simulink model "sf_cruise_control"  (Simulink 6.0)
settings: Solver=ode5  SolverMode=SingleTasking  StartTime=0.0  StopTime=inf  FixedStep=0.005  RelTol=1e-3
PreLoadFcn:
  | Kp = 30; Ki = 10; Kd = 30;
undefined symbols (not defined in the file or in its folder): DiscIntNeverNeededParam
libraries: simulink x1
CloseFcn:
  | figH = findobj('Tag','sf_cruise_control_ui'); if ~isempty(figH) delete(figH); end
settings Model: CovMetricSettings=dcmtr  CovHTMLOptions=-aTS=0 -bRG=1 -bTC=0 -hTR=0 -nFC=1  Creator=The MathWorks Inc.  LastModifiedBy=batserve  ExtModeAutoUpdateStatusClock=off
settings OptimizationCC: BooleanDataType=off
settings DebuggingCC: CheckExecutionContextPreStartOutputMsg=on  CheckExecutionContextRuntimeOutputMsg=on  SolverPrmCheckMsg=none
settings HardwareCC: TargetUnknown=on

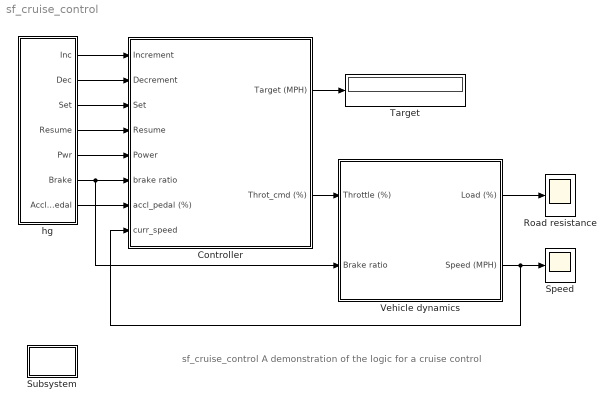
== system sf_cruise_control ==
  note: sf_cruise_control
      | A demonstration of the logic for a cruise control
  Controller : Subsystem  PropExecContextAcrossSSBoundary=on
  Road resistance : Scope
      settings: TimeRange=80  YMin=-10  YMax=40  SampleInput=on  SampleTime=0.5
  Speed : Scope
      settings: TickLabels=on  TimeRange=80  YMin=-20  YMax=100  SampleInput=on  SampleTime=0.5
  Subsystem : Subsystem  PropExecContextAcrossSSBoundary=on
      mask Display: disp('Info')
  Target : Display
  Vehicle dynamics : Subsystem  PropExecContextAcrossSSBoundary=on
  hg : Subsystem  LoadFcn=|  PropExecContextAcrossSSBoundary=on
      | figH = sf_cruise_control_ui;   
      | set_param(gcb,'UserData',figH);
      settings: AttributesFormatString=\n\n\n\n
      settings: OpenFcn=|
      | figH = get_param(gcb,'UserData');
      | if ~isempty(figH) figure(figH); end
      mask Display: disp('GUI \n Signals')
  wires:
  hg/3(Set) -> Controller/3(Set)
  hg/4(Resume) -> Controller/4(Resume)
  hg/5(Pwr) -> Controller/5(Power)
  hg/6(Brake) -> Vehicle dynamics/2(Brake ratio), Controller/6(brake ratio)
  hg/7(Accl_pedal) -> Controller/7(accl_pedal (%))
  Controller/2(Throt_cmd (%)) -> Vehicle dynamics/1(Throttle (%))
  Vehicle dynamics/2(Speed (MPH)) -> Speed/1, Controller/8(curr_speed)
  Controller/1(Target (MPH)) -> Target/1
  hg/1(Inc) -> Controller/1(Increment)
  hg/2(Dec) -> Controller/2(Decrement)
  Vehicle dynamics/1(Load (%)) -> Road resistance/1

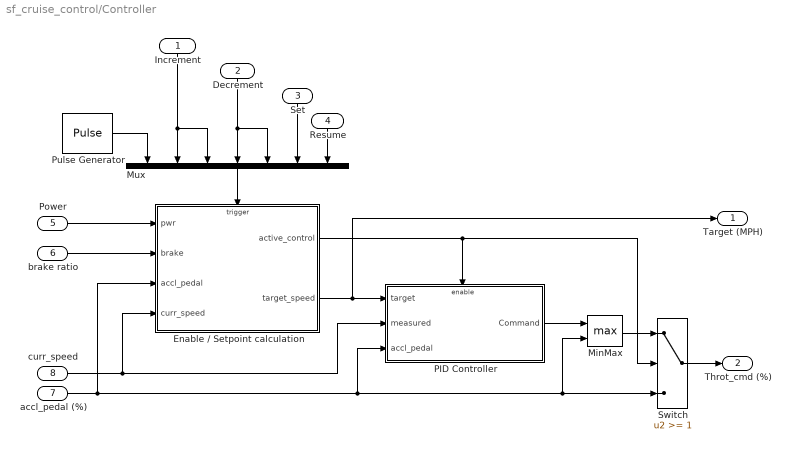
== system sf_cruise_control/Controller ==
  Increment : Inport  Orientation=down  Port=1  LatchInput=off
  Decrement : Inport  Orientation=down  Port=2  LatchInput=off
  Set : Inport  Orientation=down  Port=3  LatchInput=off
  Resume : Inport  Orientation=down  Port=4  LatchInput=off
  Power : Inport  Port=5  LatchInput=off
  brake ratio : Inport  Port=6  LatchInput=off
  accl_pedal (%) : Inport  Port=7  LatchInput=off
  curr_speed : Inport  Port=8  LatchInput=off
  Enable / Setpoint calculation : Stateflow chart  TreatAsAtomicUnit=on  PropExecContextAcrossSSBoundary=on
  MinMax : MinMax  Function=max  Inputs=2  ZeroCross=off  SaturateOnIntegerOverflow=on  InputSameDT=on
  Mux : Mux  Orientation=down  Inputs=7
  PID Controller : Subsystem  TreatAsAtomicUnit=on  PropExecContextAcrossSSBoundary=on
  Pulse Generator : DiscretePulseGenerator  SampleTime=.05
  Switch : Switch  Threshold=1  ZeroCross=off  InputSameDT=on
  Target (MPH) : Outport
  Throt_cmd (%) : Outport  Port=2
  wires:
  Pulse Generator/1 -> Mux/1
  PID Controller/1(Command) -> MinMax/1
  MinMax/1 -> Switch/1
  Enable / Setpoint calculation/1(active_control) -> PID Controller/Enable, Switch/2
  Switch/1 -> Throt_cmd (%)/1
  brake ratio/1 -> Enable / Setpoint calculation/2(brake)
  Power/1 -> Enable / Setpoint calculation/1(pwr)
  Resume/1 -> Mux/7
  Set/1 -> Mux/6
  Decrement/1 -> Mux/4, Mux/5
  Increment/1 -> Mux/2, Mux/3
  accl_pedal (%)/1 -> MinMax/2, Switch/3, PID Controller/3(accl_pedal), Enable / Setpoint calculation/3(accl_pedal)
  curr_speed/1 -> Enable / Setpoint calculation/4(curr_speed), PID Controller/2(measured)
  Enable / Setpoint calculation/2(target_speed) -> Target (MPH)/1, PID Controller/1(target)
  Mux/1 -> Enable / Setpoint calculation/Trigger

== system sf_cruise_control/Subsystem ==
  note: This model was discussed in:
      |
      | Aldrich, W. "Coverage Analysis for Model Based Design Tool",
      | Proceedings, 18th Testing Computer Software Conference, June 2001
      |
      | Available for download from
      | http://www.mathworks.com/products/simulink/technicalliterature.shtml

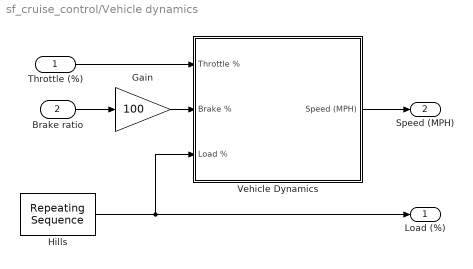
== system sf_cruise_control/Vehicle dynamics ==
  Throttle (%) : Inport  Port=1  LatchInput=off
  Brake ratio : Inport  Port=2  LatchInput=off
  Gain : Gain  Gain=100  SaturateOnIntegerOverflow=on
  Hills : simulink/Sources/Repeating Sequence  rep_seq_t=[0 2 3 5 6 8]*10  rep_seq_y=[10 15 5 20 10 -2]
  Vehicle Dynamics : Subsystem  PropExecContextAcrossSSBoundary=on
  Load (%) : Outport
  Speed (MPH) : Outport  Port=2
  wires:
  Hills/1 -> Load (%)/1, Vehicle Dynamics/3(Load %)
  Brake ratio/1 -> Gain/1
  Throttle (%)/1 -> Vehicle Dynamics/1(Throttle %)
  Vehicle Dynamics/1(Speed (MPH)) -> Speed (MPH)/1
  Gain/1 -> Vehicle Dynamics/2(Brake %)

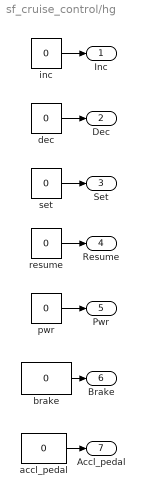
== system sf_cruise_control/hg ==
  accl_pedal : Constant  Value=0
  brake : Constant  Value=0
  dec : Constant  Value=0
  inc : Constant  Value=0
  pwr : Constant  Value=0
  resume : Constant  Value=0
  set : Constant  Value=0
  Inc : Outport
  Dec : Outport  Port=2
  Set : Outport  Port=3
  Resume : Outport  Port=4
  Pwr : Outport  Port=5
  Brake : Outport  Port=6
  Accl_pedal : Outport  Port=7
  wires:
  inc/1 -> Inc/1
  dec/1 -> Dec/1
  set/1 -> Set/1
  resume/1 -> Resume/1
  pwr/1 -> Pwr/1
  brake/1 -> Brake/1
  accl_pedal/1 -> Accl_pedal/1

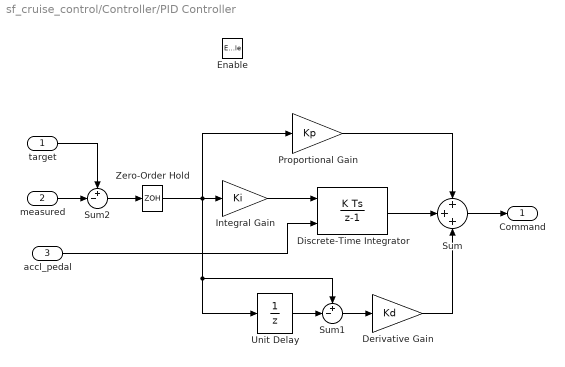
== system sf_cruise_control/Controller/PID Controller ==
  target : Inport  Port=1  LatchInput=off
  measured : Inport  Port=2  LatchInput=off
  accl_pedal : Inport  Port=3  LatchInput=off
  Enable : EnablePort  StatesWhenEnabling=reset  ZeroCross=off
  Derivative Gain : Gain  Gain=Kd  SaturateOnIntegerOverflow=on
  Discrete-Time Integrator : DiscreteIntegrator  InitialConditionSource=external  SampleTime=0.1  UpperSaturationLimit=20  LowerSaturationLimit=-20  ICPrevOutput=DiscIntNeverNeededParam  ICPrevScaledInput=DiscIntNeverNeededParam
  Integral Gain : Gain  Gain=Ki  SaturateOnIntegerOverflow=on
  Proportional Gain : Gain  Gain=Kp  SaturateOnIntegerOverflow=on
  Sum : Sum  Inputs=+++  SaturateOnIntegerOverflow=on  InputSameDT=on
  Sum1 : Sum  Inputs=+-|  SaturateOnIntegerOverflow=on  InputSameDT=on
  Sum2 : Sum  Inputs=+-|  SaturateOnIntegerOverflow=on  InputSameDT=on
  Unit Delay : UnitDelay  SampleTime=0.1
  Zero-Order Hold : ZeroOrderHold  SampleTime=0.1
  Command : Outport
  wires:
  Zero-Order Hold/1 -> Integral Gain/1, Sum1/1, Unit Delay/1, Proportional Gain/1
  accl_pedal/1 -> Discrete-Time Integrator/2
  Integral Gain/1 -> Discrete-Time Integrator/1
  measured/1 -> Sum2/2
  target/1 -> Sum2/1
  Sum/1 -> Command/1
  Sum2/1 -> Zero-Order Hold/1
  Proportional Gain/1 -> Sum/1
  Derivative Gain/1 -> Sum/3
  Discrete-Time Integrator/1 -> Sum/2
  Sum1/1 -> Derivative Gain/1
  Unit Delay/1 -> Sum1/2

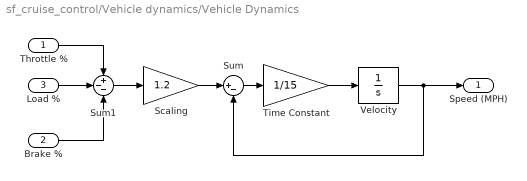
== system sf_cruise_control/Vehicle dynamics/Vehicle Dynamics ==
  Throttle % : Inport  Port=1  LatchInput=off
  Brake % : Inport  Port=2  LatchInput=off
  Load % : Inport  Port=3  LatchInput=off
  Scaling : Gain  Gain=1.2  SaturateOnIntegerOverflow=on
  Sum : Sum  Inputs=|+-  SaturateOnIntegerOverflow=on  InputSameDT=on
  Sum1 : Sum  Inputs=+--  SaturateOnIntegerOverflow=on  InputSameDT=on
  Time Constant : Gain  Gain=1/15  SaturateOnIntegerOverflow=on
  Velocity : Integrator  LimitOutput=on  LowerSaturationLimit=0  ZeroCross=off
  Speed (MPH) : Outport
  wires:
  Time Constant/1 -> Velocity/1
  Sum/1 -> Time Constant/1
  Scaling/1 -> Sum/1
  Sum1/1 -> Scaling/1
  Velocity/1 -> Speed (MPH)/1, Sum/2
  Load %/1 -> Sum1/2
  Throttle %/1 -> Sum1/1
  Brake %/1 -> Sum1/3

== stateflow chart Controller/Enable / Setpoint calculation ==
  state Set_Point_Calculation [parallel]
    state Hold
      Hold -> (junction 13) : Set [pwr]
          | {
          | target_speed = curr_speed;
          | set_speed = curr_speed;
          | }
      Hold -> (junction 14) : Resume [pwr]
      (junction 14) -> (junction 15)
      (junction 14) -> (junction 15) : [set_speed > 0]
          |
          | {target_speed = ...
          | set_speed;}
    state Increment
      en: target_speed++;
      Increment -> Increment : every(10,Update)
          | {target_speed++;}
    state Decrement
      en: target_speed--;
      Decrement -> Decrement : every(10,Update)
          | {target_speed--;}
    (default) -> Hold
    Hold -> Increment : INC_BD
        | [in(active_control)]
    Increment -> Hold : INC_BU
    Decrement -> Hold : DEC_BU
    Hold -> Decrement : DEC_BD
        | [in(active_control)]
  state Enable_logic [parallel]
    state Off
    state on
      state active_control
      state overide
        target_speed = 0;
      state no_target
      no_target -> active_control : Set
      (default) -> no_target
      active_control -> overide : [brake]
      overide -> active_control : Set | Resume
    on -> Off : [!pwr]
    Off -> on : [pwr]
    (default) -> Off
  data: pwr input boolean; brake input boolean; accl_pedal input double; active_control output State; target_speed output double; set_speed local double; curr_speed input double
  events: Update input RISING_EDGE_EVENT; INC_BD input RISING_EDGE_EVENT; INC_BU input FALLING_EDGE_EVENT; DEC_BD input RISING_EDGE_EVENT; DEC_BU input FALLING_EDGE_EVENT; Set input EITHER_EDGE_EVENT; Resume input EITHER_EDGE_EVENT
